simulink model "deadzone"  (R2023b)
settings: Solver=VariableStepAuto  StartTime=0.0  StopTime=10.0  RelTol=1e-3
settings Model: Creator=pratikmandi  LastModifiedBy=pratikmandi

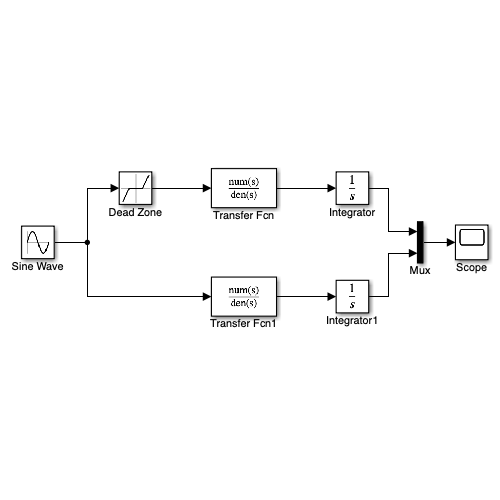
[thumbnail: Simulink's stored preview of the top-level diagram]
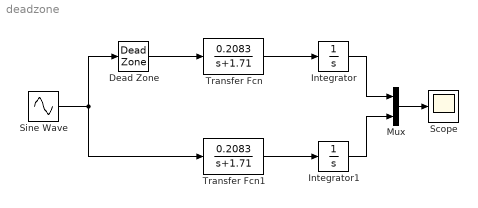
== system deadzone ==
  Dead Zone : DeadZone
  Integrator : Integrator
  Integrator1 : Integrator
  Mux : Mux  Inputs=2
  Scope : Scope
  Sine Wave : Sin  SampleTime=0
  Transfer Fcn : TransferFcn  Numerator=[0.2083]  Denominator=[1 1.71]
  Transfer Fcn1 : TransferFcn  Numerator=[0.2083]  Denominator=[1 1.71]
  wires:
  Sine Wave/1 -> Transfer Fcn1/1, Dead Zone/1
  Dead Zone/1 -> Transfer Fcn/1
  Transfer Fcn/1 -> Integrator/1
  Transfer Fcn1/1 -> Integrator1/1
  Integrator1/1 -> Mux/2
  Integrator/1 -> Mux/1
  Mux/1 -> Scope/1
